simulink model "Super2"  (Simulink 5.0)
settings: Solver=ode45  StartTime=0.0  StopTime=10.0  RelTol=1e-3
settings Model: Creator=scaife  LastModifiedBy=scaife  ExtModeAutoUpdateStatusClock=off

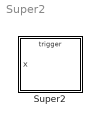
== system Super2 ==
  Super2 : Stateflow chart

== stateflow chart Super2 ==
  state A
  state B
  state C
    state C1
    (default) -> C1
  A -> C1 : E
  C1 -> B : E
  (default) -> A
  A -> C : F
  C -> B : F
  B -> A : G
  data: x input int32
  events: E input EITHER_EDGE_EVENT; F input EITHER_EDGE_EVENT; G input EITHER_EDGE_EVENT
